simulink model "pd_nf_pi_dvco"  (R2023a)
settings: configuration reference "Configuration" (kept outside this file)
values from neighbouring files (symbols this model uses):
  h_g_z : value not decoded    [dictionary_srf_pll.sldd]
  NF_z2 : value not decoded    [dictionary_srf_pll.sldd]
settings Model: DataDictionary=dictionary_srf_pll.sldd  Creator=ASUSTUF  LastModifiedBy=ASUSTUF
settings ConfigSetRef: SourceName=Configuration

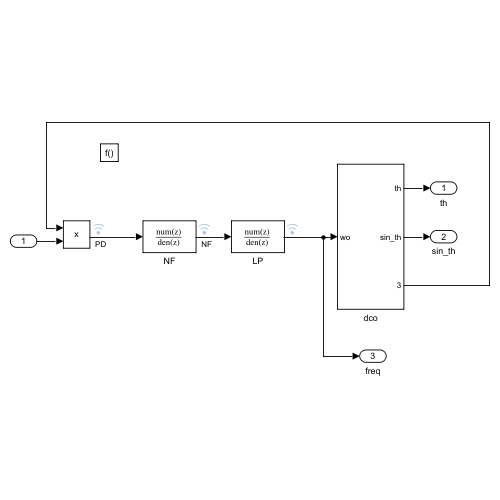
[thumbnail: Simulink's stored preview of the top-level diagram]
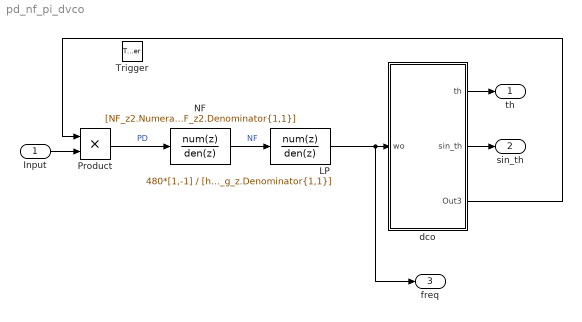
== system pd_nf_pi_dvco ==
  Input : Inport
  Trigger : TriggerPort  TriggerType=function-call  VariantControl=(inherit)  PortDimensions=1
  LP : DiscreteTransferFcn  Numerator=480*[1,-1]  Denominator=[h_g_z.Denominator{1,1}]  OutDataTypeStr=fixdt(1,32,24)
  NF : DiscreteTransferFcn  Numerator=[NF_z2.Numerator{1,1}]  Denominator=[NF_z2.Denominator{1,1}]  OutDataTypeStr=fixdt(1,32,31)
  Product : Product
  dco : Subsystem
  th : Outport
  sin_th : Outport  Port=2
  freq : Outport  Port=3
  wires:
  Input/1 -> Product/2
  NF/1 -> LP/1  "NF"
  Product/1 -> NF/1  "PD"
  LP/1 -> freq/1, dco/1(wo)
  dco/1(th) -> th/1
  dco/2(sin_th) -> sin_th/1
  dco/3(Out3) -> Product/1

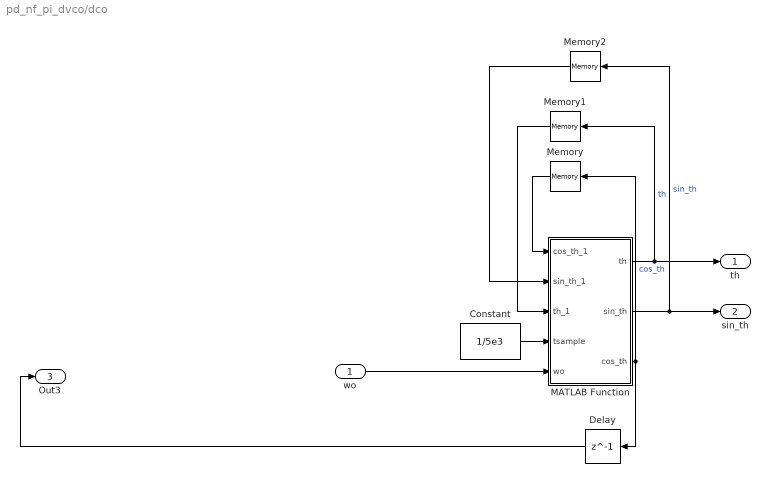
== system pd_nf_pi_dvco/dco ==
  wo : Inport
  Constant : Constant  Value=1/5e3
  Delay : Delay  DelayLength=1
  MATLAB Function : MATLAB Function  TreatAsAtomicUnit=on
  Memory : Memory  InitialCondition=.99  InheritSampleTime=on
  Memory1 : Memory  InheritSampleTime=on
  Memory2 : Memory  InheritSampleTime=on
  th : Outport
  sin_th : Outport  Port=2
  Out3 : Outport  Port=3
  wires:
  Memory/1 -> MATLAB Function/1(cos_th_1)
  MATLAB Function/1(th) -> th/1, Memory1/1  "th"
  Constant/1 -> MATLAB Function/4(tsample)
  MATLAB Function/3(cos_th) -> Memory/1, Delay/1  "cos_th"
  MATLAB Function/2(sin_th) -> sin_th/1, Memory2/1  "sin_th"
  Memory2/1 -> MATLAB Function/2(sin_th_1)
  wo/1 -> MATLAB Function/5(wo)
  Memory1/1 -> MATLAB Function/3(th_1)
  Delay/1 -> Out3/1

== matlab function pd_nf_pi_dvco/dco/MATLAB Function ==
  data: cos_th_1 input; sin_th_1 input; th_1 input; tsample input; th output; sin_th output; wo input; cos_th output
 function [th,sin_th,cos_th]= dco(cos_th_1,sin_th_1,th_1,tsample,wo)
        ws=(2*pi*50);
        wout=(wo+ws);
        
        %Sin is for showing the overlaping w the input 
        sin_th=sin_th_1+(cos_th_1*wout*tsample);%Sin(t+dt)=sin(t)+cos(t)*dt
        cos_th=cos_th_1-(sin_th_1*wout*tsample);
        
        sin_th=max([sin_th -1]);
        cos_th=max([cos_th -1]);

        sin_th=min([sin_th 1]);
        cos_th=min([cos_th 1]);

        th=th_1+(wout*tsample);

        if sin_th_1>=0 && sin_th<=0
            th=-pi;%fi(pi,1,32,29); %zero crossing reseting phase angle
        end
      
end
